simulink library "PFB_FIR"  (R2019a)
settings: Solver=VariableStepAuto  StartTime=0.0  StopTime=10.0  RelTol=1e-3
libraries: xbsIndex_r4 x1
settings Model: Creator=talonm  LastModifiedBy=mybur

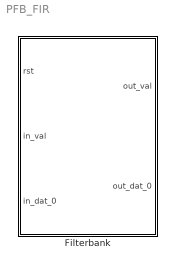
== system PFB_FIR ==
  Filterbank : Subsystem  mask{big_endian_wb_in=off, big_endian_wb_out=off, wb_factor=1, nof_chan=0, nof_bands=1024, nof_taps=4, nof_streams=1, in_dat_w=8, out_dat_w=10, coef_dat_w=12, win="hanning", fwidth=0, backoff_w=0, technology=0, ram_primitive="auto"}
      mask prompts: big_endian_wb_in "Big endian in"; big_endian_wb_out "Big endian out"; wb_factor "Wideband factor"; nof_chan "Number of Channels"; nof_bands "Number of bands"; nof_taps "Number of taps"; nof_streams "Number of streams"; in_dat_w "Input data width"; out_dat_w "Output data width"; coef_dat_w "Coefficient data width"; win "Window function"; backoff_w "Backoff width"; technology "Vendor (0-Xilinx, 1-Intel)"; ram_primitive "Ram primitive"
      mask init:
      | Simulink.Block.eval([gcb, '/filterbank_top']);
      | 
      | fil_subsys2bb_knit();
      mask TypeOptions win: "hanning" | "hamming" | "blackman" | "bartlett"
      mask TypeOptions technology: 0 | 1
      mask TypeOptions ram_primitive: "auto" | "block" | "ultra" | "distributed"

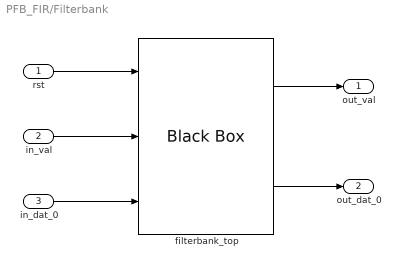
== system PFB_FIR/Filterbank ==
  rst : Inport
  in_val : Inport  Port=2
  in_dat_0 : Inport  Port=3
  filterbank_top : xbsIndex_r4/Black Box  init_code=filterbank_top_config  sim_method=ISE Simulator  verbose=off  block_type=blackbox2
  out_val : Outport
  out_dat_0 : Outport  Port=2
  wires:
  in_val/1 -> filterbank_top/2
  rst/1 -> filterbank_top/1
  in_dat_0/1 -> filterbank_top/3
  filterbank_top/1 -> out_val/1
  filterbank_top/2 -> out_dat_0/1
